simulink model "PPN"  (R2023b)
settings: Solver=ode4  StartTime=0.0  StopTime=inf  FixedStep=1/50  RelTol=1e-3
libraries: simulink x1
settings Model: Creator=sametuslu  LastModifiedBy=sametuslu

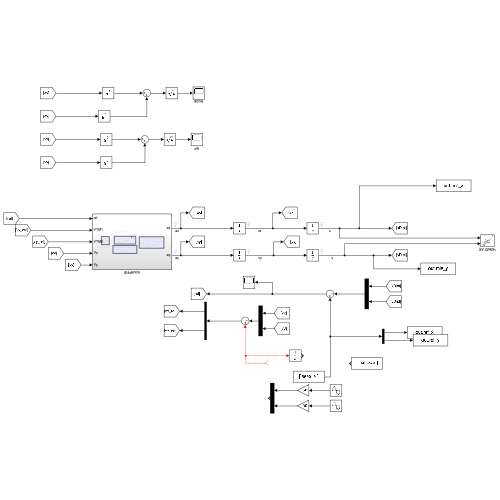
[thumbnail: Simulink's stored preview of the top-level diagram]
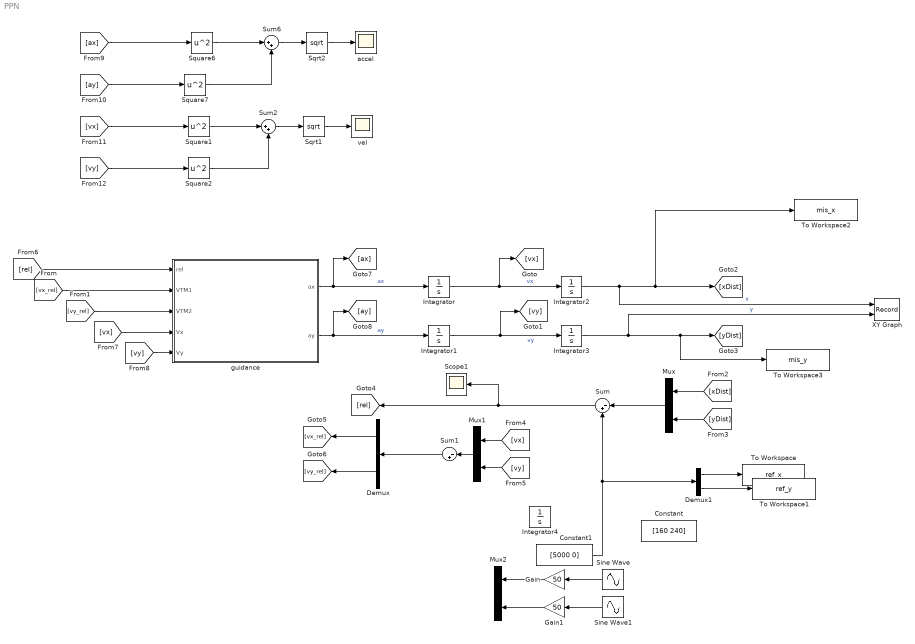
== system PPN ==
  Constant : Constant  Value=[160 240]
  Constant1 : Constant  Value=[5000 0]
  Demux : Demux  Outputs=2
  Demux1 : Demux  Outputs=2
  Gain : Gain  Gain=50
  Gain1 : Gain  Gain=50
  Integrator : Integrator  InitialCondition=200
  Integrator1 : Integrator  InitialCondition=200
  Integrator2 : Integrator
  Integrator3 : Integrator
  Integrator4 : Integrator  InitialCondition=[5000 0]
  Mux : Mux  Inputs=2
  Mux1 : Mux  Inputs=2
  Mux2 : Mux  Inputs=2
  Scope1 : Scope
  Sine Wave : Sin  Frequency=10  SampleTime=1/50
  Sine Wave1 : Sin  Frequency=10  SampleTime=1/50
  Sqrt1 : Sqrt
  Sqrt2 : Sqrt
  Square{1..2,6..7} (4 alike) : Math  Operator=square
  Sum : Sum  Inputs=|-+
  Sum1 : Sum  Inputs=|-+
  Sum2 : Sum  Inputs=|++
  Sum6 : Sum  Inputs=|++
  To Workspace : ToWorkspace  VariableName=ref_x  SampleTime=-1
  To Workspace1 : ToWorkspace  VariableName=ref_y  SampleTime=-1
  To Workspace2 : ToWorkspace  VariableName=mis_x  SampleTime=-1
  To Workspace3 : ToWorkspace  VariableName=mis_y  SampleTime=-1
  XY Graph : Record  FileSettingsInternal="{\"entries\":[{\"content\":{\"excelSettings\":{\"content\":{},\"type\":\"Streamout.ExcelSettings\"}},\"type\":\"Streamout.FileSettingStorage\",\"uuid\":\"\"}],\"packageUris\":[\"http:\\/\\/schema.mathworks.com\\/mf0\\/streamout_blocks\\/R2020a\"],\"version\":\"1.0\"}"  Layout=[1 1]  SignalsInternal="{\"entries\":[{\"content\":{\"signals\":[{\"content\":{\"blockPath\":[],\"dimensions\":[1],\"domain\":\"\",\"lineColor\":\"#a2142f\",\"plots\":[ 1 ],\"port\":1,\"sid\":[\"\"],\"signalID\":1,\"signalName\":\"x\"},\"type\":\"RecordBlkView.Signal\",\"uuid\":\"\"},{\"content\":{\"blockPath\":[],\"dimensions\":[1],\"domain\":\"\",\"lineColor\":\"#139fff\",\"plots\":[ 1 ],\"port\":2,\"sid\":[\"\"],\"signalID\":2,\"signalName\":\"y\"},\"type\":\"RecordBlkView.Signal\",\"uuid\":\"\"}]},\"type\":\"RecordBlkView.InputSignals\",\"uuid\":\"\"}],\"packageUris\":[\"http:\\/\\/schema.mathworks.com\\/mf0\\/streamout_blocks\\/R2020a\"],\"version\":\"1.0\"}"  VisualizationBindings="{\"xyplotplugin\":{\"info\":[{\"series\":[{\"bindingParametersList\":[{\"parameter\":\"X-Axis\",\"signalID\":1,\"signalName\":\"x\"},{\"parameter\":\"Y-Axis\",\"signalID\":2,\"signalName\":\"y\"}],\"seriesID\":0}],\"subplotID\":1}]}}"  CompatibilityTag=XY
  accel : Scope
  guidance : Subsystem
  vel : Scope
  wires:
  guidance/1(ax) -> Integrator/1, [ax]  "ax"
  guidance/2(ay) -> Integrator1/1, [ay]  "ay"
  Integrator/1 -> [vx], Integrator2/1  "vx"
  Integrator1/1 -> [vy], Integrator3/1  "vy"
  [vx_rel] -> guidance/2(VTM1)
  [vy_rel] -> guidance/3(VTM2)
  Integrator2/1 -> XY Graph/1, To Workspace2/1, [xDist]  "x"
  Integrator3/1 -> XY Graph/2, To Workspace3/1, [yDist]  "y"
  [xDist] -> Mux/1
  [yDist] -> Mux/2
  Mux/1 -> Sum/1
  ? -> Sum1/2, Integrator4/1
  Constant1/1 -> Demux1/1, Sum/2
  Sum/1 -> Scope1/1, [rel]
  Mux1/1 -> Sum1/1
  [vx] -> Mux1/1
  [vy] -> Mux1/2
  Sum1/1 -> Demux/1
  [rel] -> guidance/1(rel)
  Demux/1 -> [vx_rel]
  Demux/2 -> [vy_rel]
  [vx] -> guidance/4(Vx)
  [vy] -> guidance/5(Vy)
  Sqrt2/1 -> accel/1
  Square6/1 -> Sum6/1
  Square7/1 -> Sum6/2
  Sum6/1 -> Sqrt2/1
  [ax] -> Square6/1
  [ay] -> Square7/1
  [vy] -> Square2/1
  [vx] -> Square1/1
  Sum2/1 -> Sqrt1/1
  Square2/1 -> Sum2/2
  Square1/1 -> Sum2/1
  Sqrt1/1 -> vel/1
  Sine Wave/1 -> Gain/1
  Gain/1 -> Mux2/1
  Sine Wave1/1 -> Gain1/1
  Gain1/1 -> Mux2/2
  Demux1/1 -> To Workspace/1
  Demux1/2 -> To Workspace1/1

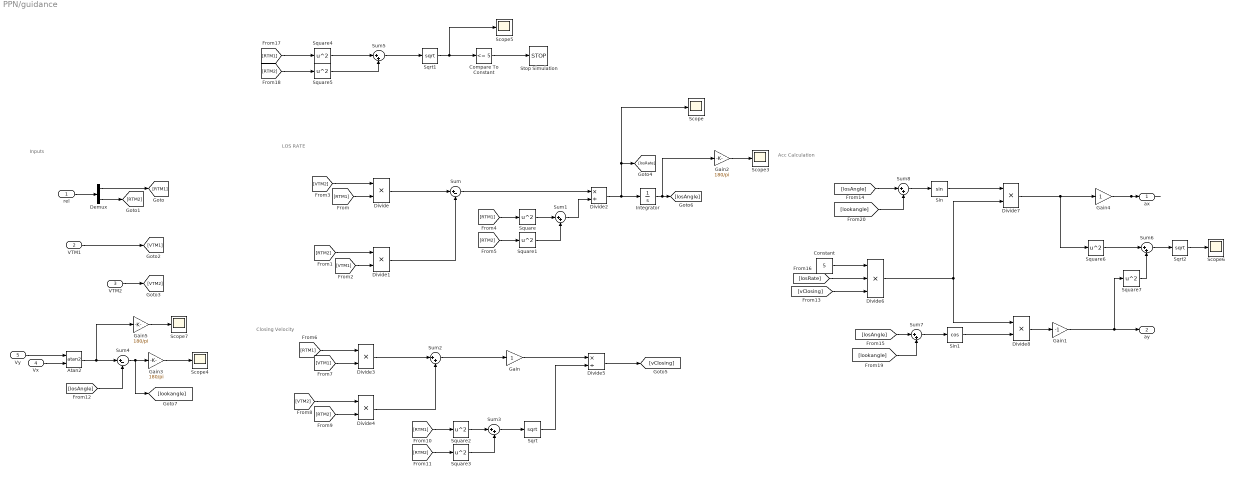
== system PPN/guidance ==
  note: Acc Calculation
  note: Closing Velocity
  note: LOS RATE
  note: Inputs
  rel : Inport
  VTM1 : Inport  Port=2
  VTM2 : Inport  Port=3
  Vx : Inport  Port=4
  Vy : Inport  Port=5
  Atan2 : Trigonometry  Operator=atan2
  Compare To Constant : simulink/Logic and Bit Operations/Compare To Constant  relop=<=  const=5  OutDataTypeStr=boolean
  Constant : Constant  Value=5
  Demux : Demux  Outputs=2
  Divide{,1,3..4,7..8} (6 alike) : Product  Inputs=**
  Divide2 : Product  Inputs=*/
  Divide5 : Product  Inputs=*/
  Divide6 : Product  Inputs=3
  Gain : Gain
  Gain1 : Gain  Gain=-1
  Gain2 : Gain  Gain=180/pi
  Gain3 : Gain  Gain=180/pi
  Gain4 : Gain
  Gain5 : Gain  Gain=180/pi
  Integrator : Integrator
  Scope{,3..7} (6 alike) : Scope
  Sin : Trigonometry
  Sin1 : Trigonometry  Operator=cos
  Sqrt : Sqrt
  Sqrt1 : Sqrt
  Sqrt2 : Sqrt
  Square{,1..7} (8 alike) : Math  Operator=square
  Stop Simulation : Stop
  Sum : Sum  Inputs=|+-
  Sum{1..3,5..8} (7 alike) : Sum  Inputs=|++
  Sum4 : Sum  Inputs=|+-
  ax : Outport
  ay : Outport  Port=2
  wires:
  rel/1 -> Demux/1
  Demux/1 -> [RTM1]
  Demux/2 -> [RTM2]
  VTM1/1 -> [VTM1]
  VTM2/1 -> [VTM2]
  [VTM2] -> Divide/1
  [RTM1] -> Divide/2
  [VTM1] -> Divide1/2
  [RTM2] -> Divide1/1
  Divide/1 -> Sum/1
  Divide1/1 -> Sum/2
  Sum/1 -> Divide2/1
  [RTM1] -> Square/1
  [RTM2] -> Square1/1
  Square/1 -> Sum1/1
  Square1/1 -> Sum1/2
  Sum1/1 -> Divide2/2
  Divide2/1 -> Scope/1, [losRate], Integrator/1
  [RTM1] -> Divide3/1
  [VTM1] -> Divide3/2
  [VTM2] -> Divide4/1
  [RTM2] -> Divide4/2
  Divide3/1 -> Sum2/1
  Divide4/1 -> Sum2/2
  Sum2/1 -> Gain/1
  Gain/1 -> Divide5/1
  Sum3/1 -> Sqrt/1
  Square3/1 -> Sum3/2
  Square2/1 -> Sum3/1
  [RTM2] -> Square3/1
  [RTM1] -> Square2/1
  Sqrt/1 -> Divide5/2
  Divide5/1 -> [vClosing]
  Integrator/1 -> Gain2/1, [losAngle]
  Constant/1 -> Divide6/1
  [losRate] -> Divide6/2
  [vClosing] -> Divide6/3
  Divide6/1 -> Divide8/1, Divide7/2
  [losAngle] -> Sum8/1
  Sin/1 -> Divide7/1
  Sin1/1 -> Divide8/2
  [losAngle] -> Sum7/1
  Divide8/1 -> Gain1/1
  Gain2/1 -> Scope3/1
  Vy/1 -> Atan2/1
  Vx/1 -> Atan2/2
  Atan2/1 -> Gain5/1, Sum4/1
  [losAngle] -> Sum4/2
  Sum4/1 -> [lookangle], Gain3/1
  Gain3/1 -> Scope4/1
  [RTM1] -> Square4/1
  [RTM2] -> Square5/1
  Square4/1 -> Sum5/1
  Square5/1 -> Sum5/2
  Sum5/1 -> Sqrt1/1
  Sqrt1/1 -> Scope5/1, Compare To Constant/1
  Compare To Constant/1 -> Stop Simulation/1
  Square6/1 -> Sum6/1
  Square7/1 -> Sum6/2
  Sum6/1 -> Sqrt2/1
  Sqrt2/1 -> Scope6/1
  Gain4/1 -> ax/1
  Gain1/1 -> Square7/1, ay/1
  Divide7/1 -> Square6/1, Gain4/1
  Gain5/1 -> Scope7/1
  Sum7/1 -> Sin1/1
  Sum8/1 -> Sin/1
  [lookangle] -> Sum7/2
  [lookangle] -> Sum8/2
